simulink model "arm_muscle"  (Simulink 8.1)
settings: Solver=ode3  StartTime=0.0  StopTime=10  FixedStep=1e-2  MaxStep=1e-2  RelTol=1e-3
values from neighbouring files (symbols this model uses):
  c = 0.05    [muscleParams.m]    (also in nms_model_MechInit.m)
  c_jointstop = 0.3 / (pi/180)    (= 17.1887338539)    [muscleParams.m]    (also in nms_model_MechInit.m)
  eref = 0.04    [muscleParams.m]    (also in nms_model_MechInit.m)
  FmaxVAS = 300    [muscleParams.m]    (also in nms_model_MechInit.m = 6000)
  g = 9.81    [init_param.m]    (also in nms_model_MechInit.m)
  K = 5    [muscleParams.m]    (also in nms_model_MechInit.m)
  L1 = 0.28    [init_param.m]
  L2 = 0.32    [init_param.m]
  loptVAS = 0.13    [muscleParams.m]    (also in nms_model_MechInit.m = 0.08)
  lslackVAS = 0.23    [muscleParams.m]    (also in nms_model_MechInit.m)
  m1 = 1.9    [init_param.m]
  N = 1.5    [muscleParams.m]    (also in nms_model_MechInit.m)
  phi23_UpLimit = 155*pi/180    (= 2.70526034059)    [muscleParams.m]    (also in nms_model_MechInit.m = 3.05432619099)
  phimaxVAS = 90*pi/180    (= 1.57079632679)    [muscleParams.m]    (also in nms_model_MechInit.m = 2.87979326579)
  phirefVAS = 60*pi/180    (= 1.0471975512)    [muscleParams.m]    (also in nms_model_MechInit.m = 2.18166156499)
  rhoVAS = 3    [muscleParams.m]    (also in nms_model_MechInit.m = 0.7)
  rVAS = 0.03    [muscleParams.m]    (also in nms_model_MechInit.m = 0.06)
  s = orProblemSendCommand(['LoadIKFastSolver robot Translation3D'],probid)    [init.m]
  tau = 0.01    [muscleParams.m]    (also in nms_model_MechInit.m)
  vmaxVAS = 12    [muscleParams.m]    (also in nms_model_MechInit.m)
  w = 0.56    [muscleParams.m]    (also in nms_model_MechInit.m)
  w_max_jointstop = 1 * pi/180    (= 0.0174532925199)    [muscleParams.m]    (also in nms_model_MechInit.m)
libraries: mblibv1 x27, simulink x1, simulink_extras x1
settings Model: Creator=hgeyer  LastModifiedBy=icoderaven
settings DataIOCC: SignalLoggingSaveFormat=Dataset
settings DebuggingCC: MultiTaskDSMMsg=warning  MultiTaskCondExecSysMsg=none  FcnCallInpInsideContextMsg=EnableAllAsWarning  StrictBusMsg=None
settings RTWCC: IncludeERTFirstTime=on
settings GRTTargetCC: CombineOutputUpdateFcns=on  GRTInterface=off
settings SimMechanicsCC: VisOnUpdateDiagram=on  VisDuringSimulation=on
settings ConfigurationSet: Description=SimMechanics 2G

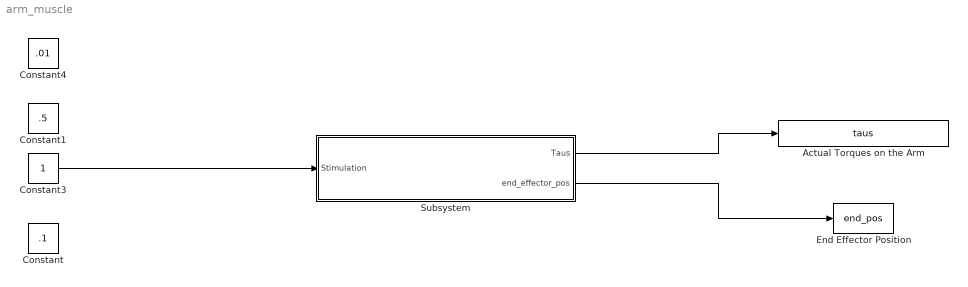
== system arm_muscle ==
  Actual Torques on the Arm : ToWorkspace  VariableName=taus  SampleTime=-1  SaveFormat=Timeseries
  Constant : Constant  Value=.1
  Constant1 : Constant  Value=.5
  Constant3 : Constant
  Constant4 : Constant  Value=.01
  End Effector Position : ToWorkspace  VariableName=end_pos  SampleTime=-1  SaveFormat=Timeseries
  Subsystem : Subsystem
  wires:
  Subsystem/1(Taus) -> Actual Torques on the Arm/1
  Subsystem/2(end_effector_pos) -> End Effector Position/1
  Constant3/1 -> Subsystem/1(Stimulation)

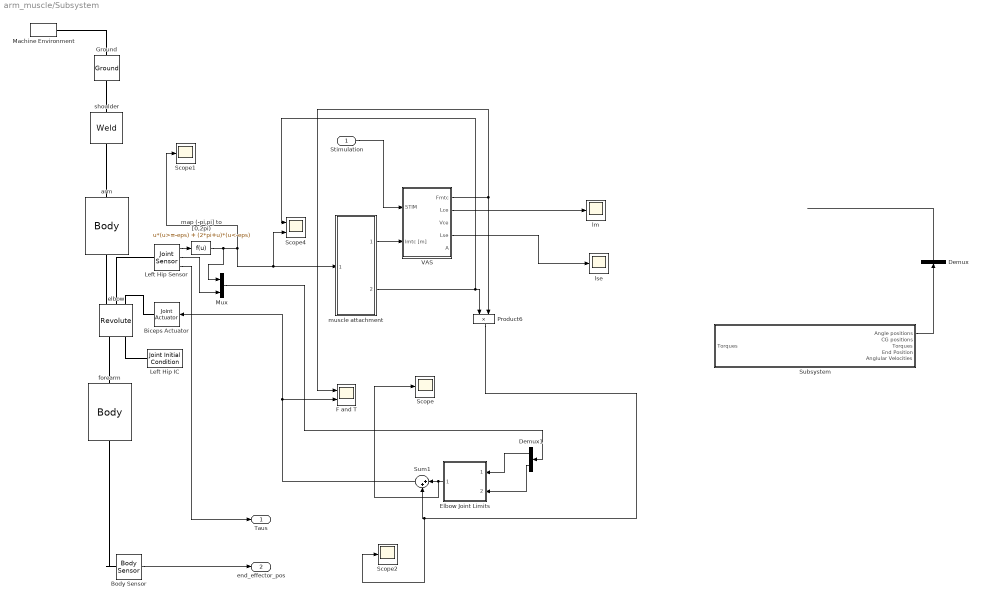
== system arm_muscle/Subsystem ==
  Stimulation : Inport
  Biceps Actuator : mblibv1/Sensors &  Actuators/Joint Actuator  UpdateFromCAD=off  PhysicalDomain=Mechanical  PortType=blob  ActuationStyle=Force  AngleUnits=deg  ArcVelocityUnits=deg/s  ArcAccelerationUnits=deg/s^2  CoordPositionUnits=m  VelocityUnits=m/s  AccelerationUnits=m/s^2  ForceUnits=N  TorqueUnits=N-m  ActiveIO=on  Width=1  DialogClass=MechanicalActuatorBlock  Primitive=R1  ReferenceFrame=Absolute (INERTIAL)
  Body Sensor : mblibv1/Sensors &  Actuators/Body Sensor  UpdateFromCAD=off  PhysicalDomain=Mechanical  PortType=blob  Muxed=on  Pose=off  Angle=on  AngleUnits=deg  ArcVelocity=off  ArcVelocityUnits=deg/s  ArcAcceleration=off  ArcAccelerationUnits=deg/s^2  CoordPosition=on  CoordPositionUnits=m  Velocity=off  VelocityUnits=m/s  Acceleration=off  AccelerationUnits=m/s^2  Quaternion=on  QuaternionDT=off  QuaternionDDT=off  QuaternionUnits=off  OutputVector=[1]  ActiveIO=on  Width=3  DialogClass=MechanicalSensorBlock  ReferenceFrame=Absolute (World)
  Demux : Demux  Outputs=3
  Demux1 : Demux  Outputs=2
  Elbow Joint Limits : Subsystem
  F and T : Scope  NumInputPorts=2
      settings: YMin=-5~-5  YMax=5~5  SaveName=ScopeData3
  Ground : mblibv1/Bodies/Ground  UpdateFromCAD=off  LeftPortType=env  RightPortType=workingframe  PhysicalDomain=Mechanical  DialogClass=GroundBlock  CoordPosition=[0 0 0]  CoordPositionUnits=m  StateVectorMgrId=3  MachineId=[4 0]  ShowEnvPort=on
  Left Hip Sensor : mblibv1/Sensors &  Actuators/Joint Sensor  UpdateFromCAD=off  PhysicalDomain=Mechanical  PortType=blob  Muxed=off  Pose=off  Angle=on  AngleUnits=rad  ArcVelocity=on  ArcVelocityUnits=rad/s  ArcAcceleration=off  ArcAccelerationUnits=deg/s^2  CoordPosition=on  CoordPositionUnits=m  Velocity=on  VelocityUnits=m/s  Acceleration=off  AccelerationUnits=m/s^2  Quaternion=on  QuaternionDT=off  QuaternionDDT=off  QuaternionUnits=off  OutputVector=[ 1 1 ]  ActiveIO=on  Width=3  DialogClass=MechanicalSensorBlock  Primitive=R1  Force=off  ForceUnits=N  Torque=on  TorqueUnits=N*m  ReferenceFrame=Absolute (INERTIAL)  ReactionSensedSide=Base  ReactionReferenceFrame=Absolute (World)  ReactionForce=off  ReactionForceUnits=N  ReactionMoment=off  ReactionMomentUnits=N*m
  Left Hip IC : mblibv1/Sensors &  Actuators/Joint Initial Condition  UpdateFromCAD=off  LeftPortType=blob  RightPortType=blob  PhysicalDomain=mechanical  DialogClass=InitialConditionBlock  InitialConditions=P1$false$0$m$rad$0$m/s$rad/s#P2$false$0$m$rad$0$m/s$rad/s#P3$false$0$m$rad$0$m/s$rad/s#R1$false$90*pi/180$m$rad$0$m/s$rad/s#R2$false$0$m$rad$0$m/s$rad/s#R3$false$0$m$rad$0$m/s$rad/s#S$false$0$m$rad$0$m/s$rad/s  P1PIC=0  P1VIC=0  P2PIC=0  P2VIC=0  P3PIC=0  P3VIC=0  R1PIC=0  R1VIC=0  R2PIC=0  R2VIC=0  R3PIC=0  R3VIC=0  SPIC=0  SVIC=0
  Machine Environment : mblibv1/Bodies/Machine Environment  PortType=env  PhysicalDomain=Mechanical  DialogTemplateClass=MECH.MachineEnvironment  SyncWhenCopied=off  Gravity=[0 -g 0]  GravityUnits=m/s^2  GravityAsSignal=off  Dimensionality=Auto-detect  AnalysisType=Forward dynamics  LinearAssemblyTolerance=1e-3  LinearAssemblyToleranceUnits=m  AngularAssemblyTolerance=1e-3  AngularAssemblyToleranceUnits=rad  ConstraintSolverType=Stabilizing  ConstraintRelTolerance=1e-4  ConstraintAbsTolerance=1e-4  UseRobustSingularityHandling=off  RedundancyAnalysisToleranceType=Automatically select tolerance  RedundancyAnalysisTolerance=1e-14  StatePerturbationType=Fixed  PerturbationSize=1e-5  VisualizeMachine=on  BodyVisualizationType=Use model default body geometries  BodyColorSelMode=Use model default  DefaultBodyColor=[1 0 0]
  Mux : Mux  Inputs=2
  Product6 : Product  RndMeth=Zero
  Scope : Scope
  Scope1 : Scope
      settings: YMin=0.588  YMax=0.5895
  Scope2 : Scope
      settings: YMin=0.588  YMax=0.5895  SaveName=ScopeData2
  Scope4 : Scope  NumInputPorts=2
      settings: YMin=-5~-5  YMax=5~5  SaveName=ScopeData4
  Subsystem : Subsystem
  Sum1 : Sum  Inputs=|++
  VAS : Subsystem
  arm : mblibv1/Bodies/Body  LConnTagsString=CS1  RConnTagsString=CS2  UpdateFromCAD=off  DialogClass=MechanicalBodyBlock  Mass=m1  MassUnits=kg  InertiaUnits=kg*m^2  Inertia=eye(3)  Shape=Cylinder  ShapeDims=[1 1]  ShapeUnits=m  ShapeUse=false  Density=1  DensityUnits=kg/m^3  DensityUse=false  GraphicsMode=MACHINE_DEFAULT  BodyColorSelMode=MACHINE_DEFAULT  BodyColor=[1 0 0]  AttachedToCS=CG  CG=Left$CG$[0 -L1 0]$CS1$CS1$m$[0 0 0]$Euler X-Y-Z$deg$WORLD$false$none  WorkingFrames=Left$CS1$[0 0 0]$Adjoining$Adjoining$m$[0 0 0]$Euler X-Y-Z$deg$WORLD$true$none#Right$CS2$[0 -L1 0]$CS1$CS1$m$[0 0 0]$Euler X-Y-Z$deg$WORLD$true$none  CGPos=[0 -L1 0]  CGRot=[0 0 0]  CS0Pos=[]  CS0Rot=[]  CS1Pos=[0 0 0]  CS1Rot=[0 0 0]  CS2Pos=[0 -L1 0]  CS2Rot=[0 0 0]  CS3Pos=[]  CS3Rot=[]  CS4Pos=[]  CS4Rot=[]  CS5Pos=[]  CS5Rot=[]  CS6Pos=[]  CS6Rot=[]  CS7Pos=[]  CS7Rot=[]  CS8Pos=[]  CS8Rot=[]  CS9Pos=[]  CS9Rot=[]  CS10Pos=[]  CS10Rot=[]  CS11Pos=[]  CS11Rot=[]  CS12Pos=[]  CS12Rot=[]  CS13Pos=[]  CS13Rot=[]  CS14Pos=[]  CS14Rot=[]  CS15Pos=[]  CS15Rot=[]  CS16Pos=[]  CS16Rot=[]  CS17Pos=[]  CS17Rot=[]  CS18Pos=[]  CS18Rot=[]  CS19Pos=[]  CS19Rot=[]  CS20Pos=[]  CS20Rot=[]
  elbow : mblibv1/Joints/Revolute  LConnTagsString=__newl0|SA1|SA2  RConnTagsString=__newr0|SA1  UpdateFromCAD=off  NumSAPorts=3  CutJoint=off  MarkAsCut=off  Primitives=prismatic  PrimitiveProps=R1$World$[0 0 1]$revolute  DialogClass=JointBlock  R1Axis=[0 0 1]
  forearm : mblibv1/Bodies/Body  LConnTagsString=CS1  RConnTagsString=CS2  UpdateFromCAD=off  DialogClass=MechanicalBodyBlock  Mass=3  MassUnits=kg  InertiaUnits=kg*m^2  Inertia=eye(3)  Shape=Cylinder  ShapeDims=[1 1]  ShapeUnits=m  ShapeUse=false  Density=1  DensityUnits=kg/m^3  DensityUse=false  GraphicsMode=MACHINE_DEFAULT  BodyColorSelMode=MACHINE_DEFAULT  BodyColor=[1 0 0]  AttachedToCS=CG  CG=Left$CG$[0 -L2 0]$CS1$CS1$m$[0 0 0]$Euler X-Y-Z$deg$WORLD$false$none  WorkingFrames=Left$CS1$[0 0 0]$Adjoining$Adjoining$m$[0 0 0]$Euler X-Y-Z$deg$WORLD$true$none#Right$CS2$[0 -L2 0]$CS1$CS1$m$[0 0 0]$Euler X-Y-Z$deg$WORLD$true$none  CGPos=[0 -L2 0]  CGRot=[0 0 0]  CS0Pos=[]  CS0Rot=[]  CS1Pos=[0 0 0]  CS1Rot=[0 0 0]  CS2Pos=[0 -L2 0]  CS2Rot=[0 0 0]  CS3Pos=[]  CS3Rot=[]  CS4Pos=[]  CS4Rot=[]  CS5Pos=[]  CS5Rot=[]  CS6Pos=[]  CS6Rot=[]  CS7Pos=[]  CS7Rot=[]  CS8Pos=[]  CS8Rot=[]  CS9Pos=[]  CS9Rot=[]  CS10Pos=[]  CS10Rot=[]  CS11Pos=[]  CS11Rot=[]  CS12Pos=[]  CS12Rot=[]  CS13Pos=[]  CS13Rot=[]  CS14Pos=[]  CS14Rot=[]  CS15Pos=[]  CS15Rot=[]  CS16Pos=[]  CS16Rot=[]  CS17Pos=[]  CS17Rot=[]  CS18Pos=[]  CS18Rot=[]  CS19Pos=[]  CS19Rot=[]  CS20Pos=[]  CS20Rot=[]
  lm : Scope
      settings: SaveName=ScopeData5
  "lse  " : Scope
      settings: TimeRange=10  SaveName=ScopeData8
  map (-pi,pi] to [0,2pi) : Fcn  Expr=u*(u>=-eps) + (2*pi+u)*(u<-eps)
  muscle attachment : Subsystem
  shoulder : mblibv1/Joints/Weld  LConnTagsString=__newl0  RConnTagsString=__newr0  UpdateFromCAD=off  NumSAPorts=0  CutJoint=off  MarkAsCut=off  Primitives=weld  PrimitiveProps=W$WORLD$[0 0 0]$weld  DialogClass=JointBlock  WAxis=[0 0 0]
  Taus : Outport
  end_effector_pos : Outport  Port=2
  wires:
  Left Hip Sensor/1 -> map (-pi,pi] to [0,2pi)/1
  muscle attachment/1(lmtu [m]) -> VAS/2(lmtc [m])
  VAS/1(Fmtc) -> F and T/1, Product6/2
  muscle attachment/2(lever [m]) -> Scope4/1, Product6/1
  Stimulation/1 -> VAS/1(STIM)
  Elbow Joint Limits/1(M_stop [Nm]) -> Scope/1, Sum1/1
  Demux1/1 -> Elbow Joint Limits/1(phi [rad])
  Demux1/2 -> Elbow Joint Limits/2(dphi [rad/s])
  Mux/1 -> Demux1/1
  Sum1/1 -> Biceps Actuator/1, F and T/2
  Product6/1 -> Scope2/1, Sum1/2
  Left Hip Sensor/2 -> Mux/2
  map (-pi,pi] to [0,2pi)/1 -> Mux/1, Scope4/2, muscle attachment/1(phi23 [rad]), Scope1/1
  Left Hip Sensor/3 -> Taus/1
  Body Sensor/1 -> end_effector_pos/1
  VAS/2(Lce) -> lm/1
  VAS/4(Lse) -> "lse  "/1
  Subsystem/1(Angle positions) -> Demux/1
  Demux/2 -> ?
  connections:
  Left Hip Sensor/LConn1 -- elbow/LConn2
  Biceps Actuator/RConn1 -- elbow/LConn3
  Machine Environment/RConn1 -- Ground/LConn1
  Ground/RConn1 -- shoulder/LConn1
  shoulder/RConn1 -- arm/LConn1
  arm/RConn1 -- elbow/LConn1
  elbow/RConn1 -- forearm/LConn1
  Left Hip IC/RConn1 -- elbow/RConn2
  Body Sensor/LConn1 -- forearm/RConn1

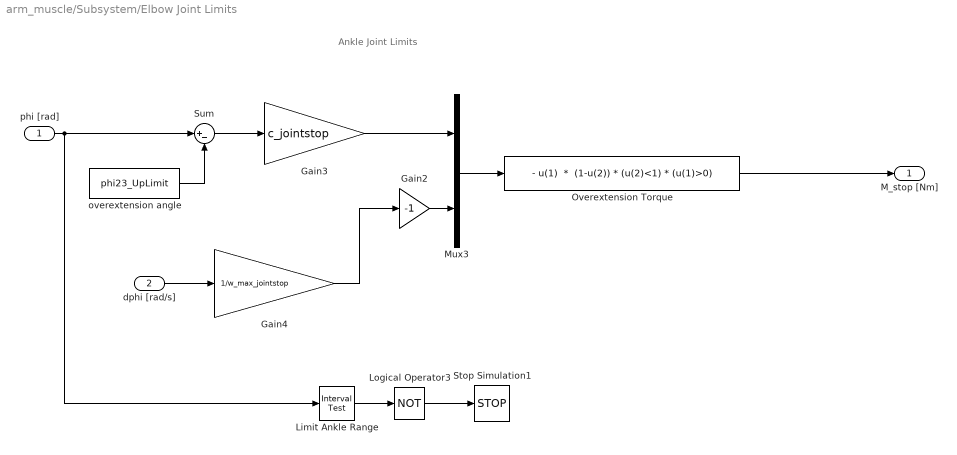
== system arm_muscle/Subsystem/Elbow Joint Limits ==
  note: Ankle Joint Limits
  phi [rad] : Inport
  dphi [rad/s] : Inport  Port=2
  Gain2 : Gain  Gain=-1
  Gain3 : Gain  Gain=c_jointstop
  Gain4 : Gain  Gain=1/w_max_jointstop
  Limit Ankle Range : simulink/Logic and Bit Operations/Interval Test  IntervalClosedRight=on  uplimit=160*pi/180  IntervalClosedLeft=on  lowlimit=0*pi/180  OutDataTypeStr=boolean
  Logical Operator3 : Logic  Operator=NOT  AllPortsSameDT=off  OutDataTypeStr=boolean
  Mux3 : Mux  Inputs=2
  Overextension Torque : Fcn  Expr="- u(1)  *  (1-u(2)) * (u(2)<1) * (u(1)>0)"
  Stop Simulation1 : Stop
  Sum : Sum  Inputs=|+-
  overextension angle : Constant  Value=phi23_UpLimit
  M_stop [Nm] : Outport
  wires:
  Mux3/1 -> Overextension Torque/1
  Gain3/1 -> Mux3/1
  dphi [rad/s]/1 -> Gain4/1
  overextension angle/1 -> Sum/2
  phi [rad]/1 -> Sum/1, Limit Ankle Range/1
  Sum/1 -> Gain3/1
  Gain4/1 -> Gain2/1
  Gain2/1 -> Mux3/2
  Overextension Torque/1 -> M_stop [Nm]/1
  Limit Ankle Range/1 -> Logical Operator3/1
  Logical Operator3/1 -> Stop Simulation1/1

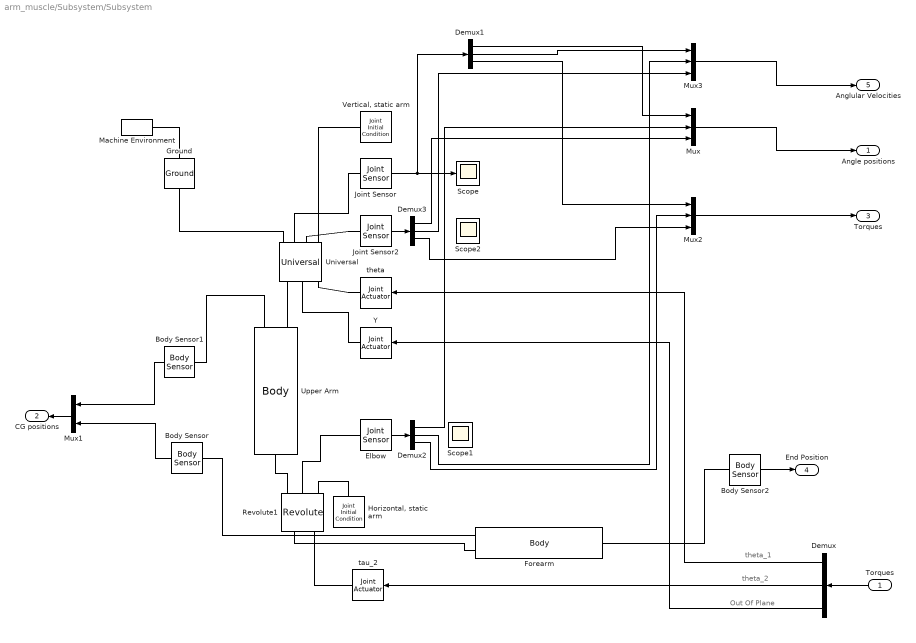
== system arm_muscle/Subsystem/Subsystem ==
  note: theta_2
  note: theta_1
  note: Out Of Plane
  "Torques " : Inport
  Body Sensor : mblibv1/Sensors &  Actuators/Body Sensor  UpdateFromCAD=off  PhysicalDomain=Mechanical  PortType=blob  Muxed=on  Pose=off  Angle=on  AngleUnits=deg  ArcVelocity=off  ArcVelocityUnits=deg/s  ArcAcceleration=off  ArcAccelerationUnits=deg/s^2  CoordPosition=on  CoordPositionUnits=m  Velocity=off  VelocityUnits=m/s  Acceleration=off  AccelerationUnits=m/s^2  Quaternion=on  QuaternionDT=off  QuaternionDDT=off  QuaternionUnits=off  OutputVector=[1]  ActiveIO=off  Width=3  DialogClass=MechanicalSensorBlock  ReferenceFrame=Absolute (World)
  Body Sensor1 : mblibv1/Sensors &  Actuators/Body Sensor  UpdateFromCAD=off  PhysicalDomain=Mechanical  PortType=blob  Muxed=on  Pose=off  Angle=on  AngleUnits=deg  ArcVelocity=off  ArcVelocityUnits=deg/s  ArcAcceleration=off  ArcAccelerationUnits=deg/s^2  CoordPosition=on  CoordPositionUnits=m  Velocity=off  VelocityUnits=m/s  Acceleration=off  AccelerationUnits=m/s^2  Quaternion=on  QuaternionDT=off  QuaternionDDT=off  QuaternionUnits=off  OutputVector=[1]  ActiveIO=off  Width=3  DialogClass=MechanicalSensorBlock  ReferenceFrame=Absolute (World)
  Body Sensor2 : mblibv1/Sensors &  Actuators/Body Sensor  UpdateFromCAD=off  PhysicalDomain=Mechanical  PortType=blob  Muxed=on  Pose=off  Angle=on  AngleUnits=deg  ArcVelocity=off  ArcVelocityUnits=deg/s  ArcAcceleration=off  ArcAccelerationUnits=deg/s^2  CoordPosition=on  CoordPositionUnits=m  Velocity=off  VelocityUnits=m/s  Acceleration=off  AccelerationUnits=m/s^2  Quaternion=on  QuaternionDT=off  QuaternionDDT=off  QuaternionUnits=off  OutputVector=[1]  ActiveIO=off  Width=3  DialogClass=MechanicalSensorBlock  ReferenceFrame=Absolute (World)
  Demux{,1..3} (4 alike) : Demux  Outputs=3
  Elbow : mblibv1/Sensors &  Actuators/Joint Sensor  UpdateFromCAD=off  PhysicalDomain=Mechanical  PortType=blob  Muxed=on  Pose=off  Angle=on  AngleUnits=rad  ArcVelocity=on  ArcVelocityUnits=rad/s  ArcAcceleration=off  ArcAccelerationUnits=deg/s^2  CoordPosition=on  CoordPositionUnits=m  Velocity=off  VelocityUnits=m/s  Acceleration=off  AccelerationUnits=m/s^2  Quaternion=on  QuaternionDT=off  QuaternionDDT=off  QuaternionUnits=off  OutputVector=[1]  ActiveIO=off  Width=3  DialogClass=MechanicalSensorBlock  Primitive=R1  Force=off  ForceUnits=N  Torque=on  TorqueUnits=N*m  ReferenceFrame=Absolute (World)  ReactionSensedSide=Base  ReactionReferenceFrame=Absolute (World)  ReactionForce=off  ReactionForceUnits=N  ReactionMoment=off  ReactionMomentUnits=N*m
  Forearm : mblibv1/Bodies/Body  LConnTagsString=CG|CS1  RConnTagsString=CS2  UpdateFromCAD=off  DialogClass=MechanicalBodyBlock  Mass=1  MassUnits=kg  InertiaUnits=kg*m^2  Inertia=eye(3)  Shape=Cylinder  ShapeDims=[1 1]  ShapeUnits=m  ShapeUse=false  Density=1  DensityUnits=kg/m^3  DensityUse=false  GraphicsMode=MACHINE_DEFAULT  BodyColorSelMode=MACHINE_DEFAULT  BodyColor=[1 0 0]  AttachedToCS=CG  CG=Left$CG$[0 -L2/2 0]$CS1$CS1$m$[0 0 0]$Euler X-Y-Z$deg$WORLD$true$none  WorkingFrames=Left$CS1$[0 0 0]$Adjoining$Adjoining$m$[0 0 0]$Euler X-Y-Z$deg$WORLD$true$none#Right$CS2$[0 -L2 0]$CS1$CS1$m$[0 0 0]$Euler X-Y-Z$deg$WORLD$true$none  CGPos=[0 -L2/2 0]  CGRot=[0 0 0]  CS0Pos=[]  CS0Rot=[]  CS1Pos=[0 0 0]  CS1Rot=[0 0 0]  CS2Pos=[0 -L2 0]  CS2Rot=[0 0 0]  CS3Pos=[]  CS3Rot=[]  CS4Pos=[]  CS4Rot=[]  CS5Pos=[]  CS5Rot=[]  CS6Pos=[]  CS6Rot=[]  CS7Pos=[]  CS7Rot=[]  CS8Pos=[]  CS8Rot=[]  CS9Pos=[]  CS9Rot=[]  CS10Pos=[]  CS10Rot=[]  CS11Pos=[]  CS11Rot=[]  CS12Pos=[]  CS12Rot=[]  CS13Pos=[]  CS13Rot=[]  CS14Pos=[]  CS14Rot=[]  CS15Pos=[]  CS15Rot=[]  CS16Pos=[]  CS16Rot=[]  CS17Pos=[]  CS17Rot=[]  CS18Pos=[]  CS18Rot=[]  CS19Pos=[]  CS19Rot=[]  CS20Pos=[]  CS20Rot=[]
  Ground : mblibv1/Bodies/Ground  UpdateFromCAD=off  LeftPortType=env  RightPortType=workingframe  PhysicalDomain=Mechanical  DialogClass=GroundBlock  CoordPosition=[0 0 0]  CoordPositionUnits=m  StateVectorMgrId=-1  MachineId=[0 0]  ShowEnvPort=on
  "Horizontal, static arm" : mblibv1/Sensors &  Actuators/Joint Initial Condition  UpdateFromCAD=off  LeftPortType=blob  RightPortType=blob  PhysicalDomain=mechanical  DialogClass=InitialConditionBlock  InitialConditions=P1$false$0$m$deg$0$m/s$deg/s#P2$false$0$m$deg$0$m/s$deg/s#P3$false$0$m$deg$0$m/s$deg/s#R1$false$0$m$deg$0$m/s$deg/s#R2$false$0$m$deg$0$m/s$deg/s#R3$false$0$m$deg$0$m/s$deg/s#S$false$0$m$deg$0$m/s$deg/s  P1PIC=0  P1VIC=0  P2PIC=0  P2VIC=0  P3PIC=0  P3VIC=0  R1PIC=0  R1VIC=0  R2PIC=0  R2VIC=0  R3PIC=0  R3VIC=0  SPIC=0  SVIC=0
  Joint Sensor : mblibv1/Sensors &  Actuators/Joint Sensor  UpdateFromCAD=off  PhysicalDomain=Mechanical  PortType=blob  Muxed=on  Pose=off  Angle=on  AngleUnits=rad  ArcVelocity=on  ArcVelocityUnits=rad/s  ArcAcceleration=off  ArcAccelerationUnits=deg/s^2  CoordPosition=on  CoordPositionUnits=m  Velocity=off  VelocityUnits=m/s  Acceleration=off  AccelerationUnits=m/s^2  Quaternion=on  QuaternionDT=off  QuaternionDDT=off  QuaternionUnits=off  OutputVector=[1]  ActiveIO=off  Width=3  DialogClass=MechanicalSensorBlock  Primitive=R1  Force=off  ForceUnits=N  Torque=on  TorqueUnits=N*m  ReferenceFrame=Absolute (World)  ReactionSensedSide=Base  ReactionReferenceFrame=Absolute (World)  ReactionForce=off  ReactionForceUnits=N  ReactionMoment=off  ReactionMomentUnits=N*m
  Joint Sensor2 : mblibv1/Sensors &  Actuators/Joint Sensor  UpdateFromCAD=off  PhysicalDomain=Mechanical  PortType=blob  Muxed=on  Pose=off  Angle=on  AngleUnits=rad  ArcVelocity=on  ArcVelocityUnits=rad/s  ArcAcceleration=off  ArcAccelerationUnits=deg/s^2  CoordPosition=on  CoordPositionUnits=m  Velocity=off  VelocityUnits=m/s  Acceleration=off  AccelerationUnits=m/s^2  Quaternion=on  QuaternionDT=off  QuaternionDDT=off  QuaternionUnits=off  OutputVector=[1]  ActiveIO=off  Width=3  DialogClass=MechanicalSensorBlock  Primitive=R2  Force=off  ForceUnits=N  Torque=on  TorqueUnits=N*m  ReferenceFrame=Absolute (World)  ReactionSensedSide=Base  ReactionReferenceFrame=Absolute (World)  ReactionForce=off  ReactionForceUnits=N  ReactionMoment=off  ReactionMomentUnits=N*m
  Machine Environment : mblibv1/Bodies/Machine Environment  PortType=env  PhysicalDomain=Mechanical  DialogTemplateClass=MECH.MachineEnvironment  SyncWhenCopied=off  Gravity=[0 -g 0]  GravityUnits=m/s^2  GravityAsSignal=off  Dimensionality=Auto-detect  AnalysisType=Forward dynamics  LinearAssemblyTolerance=1e-3  LinearAssemblyToleranceUnits=m  AngularAssemblyTolerance=1e-3  AngularAssemblyToleranceUnits=rad  ConstraintSolverType=Stabilizing  ConstraintRelTolerance=1e-4  ConstraintAbsTolerance=1e-4  UseRobustSingularityHandling=off  RedundancyAnalysisToleranceType=Automatically select tolerance  RedundancyAnalysisTolerance=1e-14  StatePerturbationType=Fixed  PerturbationSize=1e-5  VisualizeMachine=on  BodyVisualizationType=Use model default body geometries  BodyColorSelMode=Use model default  DefaultBodyColor=[1 0 0]
  Mux : Mux  Inputs=3
  Mux1 : Mux  Inputs=2
  Mux2 : Mux  Inputs=3
  Mux3 : Mux  Inputs=3
  Revolute1 : mblibv1/Joints/Revolute  LConnTagsString=__newl0|SA1|SA2  RConnTagsString=__newr0|SA1  UpdateFromCAD=off  NumSAPorts=3  CutJoint=off  MarkAsCut=off  Primitives=prismatic  PrimitiveProps=R1$World$[0 0 1]$revolute  DialogClass=JointBlock  R1Axis=[0 0 1]
  Scope : Scope
  Scope1 : Scope
  Scope2 : Scope
      settings: SaveName=ScopeData2
  Universal : mblibv1/Joints/Universal  LConnTagsString=__newl0|SA1|SA2|SA3  RConnTagsString=__newr0|SA1|SA2  UpdateFromCAD=off  NumSAPorts=5  CutJoint=off  MarkAsCut=off  Primitives=prismatic  PrimitiveProps=R1$World$[0 0 1]$revolute#R2$World$[1 0 0]$revolute  DialogClass=JointBlock  R1Axis=[0 0 1]  R2Axis=[1 0 0]
  Upper Arm : mblibv1/Bodies/Body  LConnTagsString=CG|CS1  RConnTagsString=CS2  UpdateFromCAD=off  DialogClass=MechanicalBodyBlock  Mass=1  MassUnits=kg  InertiaUnits=kg*m^2  Inertia=eye(3)  Shape=Cylinder  ShapeDims=[1 1]  ShapeUnits=m  ShapeUse=false  Density=1  DensityUnits=kg/m^3  DensityUse=false  GraphicsMode=MACHINE_DEFAULT  BodyColorSelMode=MACHINE_DEFAULT  BodyColor=[1 0 0]  AttachedToCS=CG  CG=Left$CG$[0 -L1/2 0]$CS1$CS1$m$[0 0 0]$Euler X-Y-Z$deg$WORLD$true$none  WorkingFrames=Left$CS1$[0 0 0]$World$World$m$[0 0 0]$Euler X-Y-Z$deg$WORLD$true$none#Right$CS2$[0 -L1 0]$CS1$CS1$m$[0 0 0]$Euler X-Y-Z$deg$WORLD$true$none  CGPos=[0 -L1/2 0]  CGRot=[0 0 0]  CS0Pos=[]  CS0Rot=[]  CS1Pos=[0 0 0]  CS1Rot=[0 0 0]  CS2Pos=[0 -L1 0]  CS2Rot=[0 0 0]  CS3Pos=[]  CS3Rot=[]  CS4Pos=[]  CS4Rot=[]  CS5Pos=[]  CS5Rot=[]  CS6Pos=[]  CS6Rot=[]  CS7Pos=[]  CS7Rot=[]  CS8Pos=[]  CS8Rot=[]  CS9Pos=[]  CS9Rot=[]  CS10Pos=[]  CS10Rot=[]  CS11Pos=[]  CS11Rot=[]  CS12Pos=[]  CS12Rot=[]  CS13Pos=[]  CS13Rot=[]  CS14Pos=[]  CS14Rot=[]  CS15Pos=[]  CS15Rot=[]  CS16Pos=[]  CS16Rot=[]  CS17Pos=[]  CS17Rot=[]  CS18Pos=[]  CS18Rot=[]  CS19Pos=[]  CS19Rot=[]  CS20Pos=[]  CS20Rot=[]
  "Vertical, static arm" : mblibv1/Sensors &  Actuators/Joint Initial Condition  UpdateFromCAD=off  LeftPortType=blob  RightPortType=blob  PhysicalDomain=mechanical  DialogClass=InitialConditionBlock  InitialConditions=P1$false$0$m$deg$0$m/s$deg/s#P2$false$0$m$deg$0$m/s$deg/s#P3$false$0$m$deg$0$m/s$deg/s#R1$true$0$m$deg$0$m/s$deg/s#R2$true$0$m$deg$0$m/s$deg/s#R3$false$0$m$deg$0$m/s$deg/s#S$false$0$m$deg$0$m/s$deg/s  P1PIC=0  P1VIC=0  P2PIC=0  P2VIC=0  P3PIC=0  P3VIC=0  R1PIC=0  R1VIC=0  R2PIC=0  R2VIC=0  R3PIC=0  R3VIC=0  SPIC=0  SVIC=0
  Y : mblibv1/Sensors &  Actuators/Joint Actuator  UpdateFromCAD=off  PhysicalDomain=Mechanical  PortType=blob  ActuationStyle=Force  AngleUnits=deg  ArcVelocityUnits=deg/s  ArcAccelerationUnits=deg/s^2  CoordPositionUnits=m  VelocityUnits=m/s  AccelerationUnits=m/s^2  ForceUnits=N  TorqueUnits=N*m  ActiveIO=off  Width=1  DialogClass=MechanicalActuatorBlock  Primitive=R2  ReferenceFrame=Absolute (World)
  tau_2 : mblibv1/Sensors &  Actuators/Joint Actuator  UpdateFromCAD=off  PhysicalDomain=Mechanical  PortType=blob  ActuationStyle=Force  AngleUnits=deg  ArcVelocityUnits=deg/s  ArcAccelerationUnits=deg/s^2  CoordPositionUnits=m  VelocityUnits=m/s  AccelerationUnits=m/s^2  ForceUnits=N  TorqueUnits=N*m  ActiveIO=off  Width=1  DialogClass=MechanicalActuatorBlock  Primitive=R1  ReferenceFrame=Absolute (World)
  theta : mblibv1/Sensors &  Actuators/Joint Actuator  UpdateFromCAD=off  PhysicalDomain=Mechanical  PortType=blob  ActuationStyle=Force  AngleUnits=deg  ArcVelocityUnits=deg/s  ArcAccelerationUnits=deg/s^2  CoordPositionUnits=m  VelocityUnits=m/s  AccelerationUnits=m/s^2  ForceUnits=N  TorqueUnits=N*m  ActiveIO=off  Width=1  DialogClass=MechanicalActuatorBlock  Primitive=R1  ReferenceFrame=Absolute (World)
  Angle positions : Outport
  "CG positions " : Outport  Port=2
  Torques : Outport  Port=3
  End Position : Outport  Port=4
  Anglular Velocities : Outport  Port=5
  wires:
  Demux/3 -> Y/1
  Demux/2 -> tau_2/1
  Joint Sensor/1 -> Demux1/1, Scope/1
  Demux/1 -> theta/1
  "Torques "/1 -> Demux/1
  Mux/1 -> Angle positions/1
  Demux1/1 -> Mux/1
  Demux2/1 -> Mux/2
  Demux3/1 -> Mux/3
  Body Sensor/1 -> Mux1/2
  Mux1/1 -> "CG positions "/1
  Body Sensor1/1 -> Mux1/1
  Mux2/1 -> Torques/1
  Demux2/3 -> Mux2/2
  Demux3/3 -> Mux2/3
  Body Sensor2/1 -> End Position/1
  Demux1/3 -> Mux2/1
  Elbow/1 -> Demux2/1
  Joint Sensor2/1 -> Demux3/1
  Mux3/1 -> Anglular Velocities/1
  Demux1/2 -> Mux3/1
  Demux3/2 -> Mux3/3
  Demux2/2 -> Mux3/2
  connections:
  Universal/LConn1 -- Ground/RConn1
  Universal/RConn1 -- Upper Arm/LConn2
  Revolute1/LConn1 -- Upper Arm/RConn1
  Revolute1/RConn1 -- Forearm/LConn2
  Machine Environment/RConn1 -- Ground/LConn1
  Universal/LConn2 -- Joint Sensor/LConn1
  Universal/RConn2 -- Y/RConn1
  tau_2/RConn1 -- Revolute1/RConn2
  Elbow/LConn1 -- Revolute1/LConn2
  theta/RConn1 -- Universal/RConn3
  Joint Sensor2/LConn1 -- Universal/LConn3
  "Vertical, static arm"/RConn1 -- Universal/LConn4
  Revolute1/LConn3 -- "Horizontal, static arm"/RConn1
  Body Sensor/LConn1 -- Forearm/LConn1
  Upper Arm/LConn1 -- Body Sensor1/LConn1
  Body Sensor2/LConn1 -- Forearm/RConn1

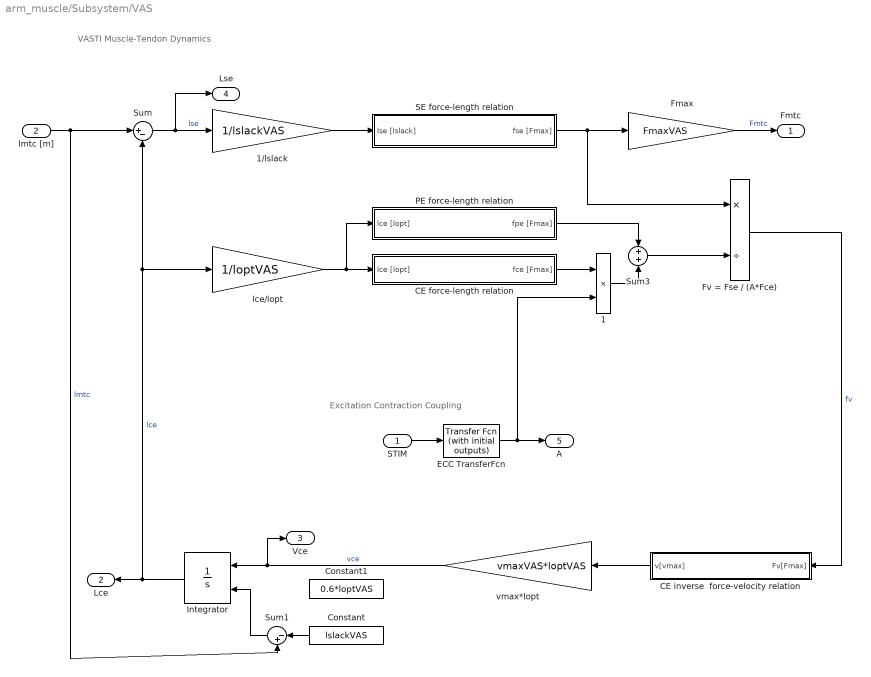
== system arm_muscle/Subsystem/VAS ==
  note: VASTI Muscle-Tendon Dynamics
  note: Excitation Contraction Coupling
  STIM : Inport
  lmtc [m] : Inport  Port=2
  1 : Product  Inputs=**  SaturateOnIntegerOverflow=on  InputSameDT=on  OutDataTypeStr=Inherit: Same as first input
  1/lslack : Gain  Gain=1/lslackVAS  SaturateOnIntegerOverflow=on  OutDataTypeStr=Inherit: Same as input  ParamDataTypeStr=Inherit: Same as input
  CE force-length relation : Subsystem
  CE inverse  force-velocity relation : Subsystem
  Constant : Constant  Value=lslackVAS
  Constant1 : Constant  Value=0.6*loptVAS
  ECC TransferFcn : simulink_extras/Additional Linear/Transfer Fcn (with initial outputs)  N=[1]  D="[tau  1]"  Y0=preA  U0=0
      settings: AttributesFormatString=pre-activation: %<Y0>
  Fmax : Gain  Gain=FmaxVAS  SaturateOnIntegerOverflow=on  OutDataTypeStr=Inherit: Same as input  ParamDataTypeStr=Inherit: Same as input
  Fv = Fse / (A*Fce) : Product  Inputs=*/  SaturateOnIntegerOverflow=on  InputSameDT=on  OutDataTypeStr=Inherit: Same as first input
  Integrator : Integrator  InitialConditionSource=external  LowerSaturationLimit=0.05
  PE force-length relation : Subsystem
  SE force-length relation : Subsystem
  Sum : Sum  Inputs=|+-  SaturateOnIntegerOverflow=on  InputSameDT=on  OutDataTypeStr=Inherit: Same as first input
  Sum1 : Sum  Inputs=|-+  SaturateOnIntegerOverflow=on  InputSameDT=on  OutDataTypeStr=Inherit: Same as first input
  Sum3 : Sum  SaturateOnIntegerOverflow=on  InputSameDT=on  OutDataTypeStr=Inherit: Same as first input
  lce/lopt : Gain  Gain=1/loptVAS  SaturateOnIntegerOverflow=on  OutDataTypeStr=Inherit: Same as input  ParamDataTypeStr=Inherit: Same as input
  vmax*lopt : Gain  Gain=vmaxVAS*loptVAS  SaturateOnIntegerOverflow=on  OutDataTypeStr=Inherit: Same as input  ParamDataTypeStr=Inherit: Same as input
  Fmtc : Outport  InitialOutput=0
  Lce : Outport  Port=2  InitialOutput=0
  Vce : Outport  Port=3  InitialOutput=0
  Lse : Outport  Port=4  InitialOutput=0
  A : Outport  Port=5  InitialOutput=0
  wires:
  Integrator/1 -> Sum/2, lce/lopt/1, Lce/1  "lce"
  Sum/1 -> 1/lslack/1, Lse/1  "lse"
  lce/lopt/1 -> CE force-length relation/1(lce [lopt]), PE force-length relation/1(lce [lopt])
  Fv = Fse / (A*Fce)/1 -> CE inverse  force-velocity relation/1(Fv[Fmax])  "fv"
  vmax*lopt/1 -> Integrator/1, Vce/1  "vce"
  lmtc [m]/1 -> Sum1/2, Sum/1  "lmtc"
  Fmax/1 -> Fmtc/1  "Fmtc"
  1/lslack/1 -> SE force-length relation/1(lse [lslack])
  Constant/1 -> Sum1/1
  CE force-length relation/1(fce [Fmax]) -> 1/1
  SE force-length relation/1(fse [Fmax]) -> Fv = Fse / (A*Fce)/1, Fmax/1
  PE force-length relation/1(fpe [Fmax]) -> Sum3/1
  1/1 -> Sum3/2
  Sum3/1 -> Fv = Fse / (A*Fce)/2
  CE inverse  force-velocity relation/1(v[vmax]) -> vmax*lopt/1
  STIM/1 -> ECC TransferFcn/1
  ECC TransferFcn/1 -> 1/2, A/1
  Sum1/1 -> Integrator/2

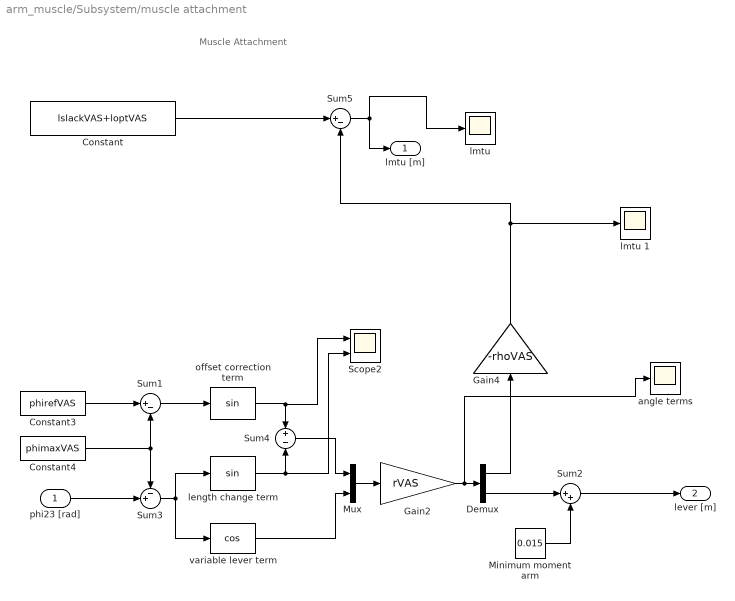
== system arm_muscle/Subsystem/muscle attachment ==
  note: Muscle Attachment
  phi23 [rad] : Inport
  Constant : Constant  Value=lslackVAS+loptVAS
  Constant3 : Constant  Value=phirefVAS
  Constant4 : Constant  Value=phimaxVAS
  Demux : Demux  Outputs=2
  Gain2 : Gain  Gain=rVAS
  Gain4 : Gain  Gain=-rhoVAS
  Minimum moment arm : Constant  Value=0.015
  Mux : Mux  Inputs=2
  Scope2 : Scope  NumInputPorts=2
      settings: YMin=0.906308~-0.9  YMax=0.906308~0.5  SaveName=ScopeData7
  Sum1 : Sum  Inputs=|+-
  Sum2 : Sum  Inputs=|++
  Sum3 : Sum  Inputs=-+|
  Sum4 : Sum  Inputs=+-
  Sum5 : Sum  Inputs=|+-
  "angle terms " : Scope
      settings: TimeRange=8  YMin=-0.03  YMax=0.03  SaveName=ScopeData6
  length change term : Trigonometry
  "lmtu " : Scope
      settings: TimeRange=4  SaveName=ScopeData5
  lmtu 1 : Scope
      settings: SaveName=ScopeData9
  offset correction term : Trigonometry
  variable lever term : Trigonometry  Operator=cos
  lmtu [m] : Outport
  lever [m] : Outport  Port=2
  wires:
  Constant/1 -> Sum5/1
  Sum5/1 -> "lmtu "/1, lmtu [m]/1
  Gain4/1 -> Sum5/2, lmtu 1/1
  phi23 [rad]/1 -> Sum3/2
  Sum3/1 -> variable lever term/1, length change term/1
  Constant4/1 -> Sum3/1, Sum1/2
  Sum1/1 -> offset correction term/1
  Constant3/1 -> Sum1/1
  offset correction term/1 -> Scope2/1, Sum4/1
  length change term/1 -> Sum4/2, Scope2/2
  variable lever term/1 -> Mux/2
  Mux/1 -> Gain2/1
  Gain2/1 -> "angle terms "/1, Demux/1
  Demux/1 -> Gain4/1
  Demux/2 -> Sum2/1
  Minimum moment arm/1 -> Sum2/2
  Sum2/1 -> lever [m]/1
  Sum4/1 -> Mux/1

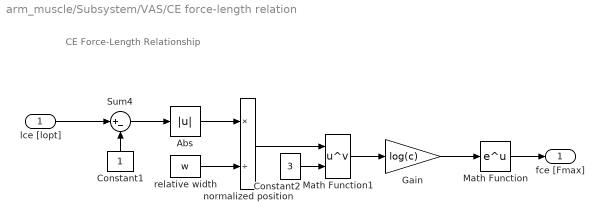
== system arm_muscle/Subsystem/VAS/CE force-length relation ==
  note: CE Force-Length Relationship
  lce [lopt] : Inport
  Abs : Abs
  Constant1 : Constant
  Constant2 : Constant  Value=3
  Gain : Gain  Gain=log(c)
  Math Function : Math  SaturateOnIntegerOverflow=on
  Math Function1 : Math  Operator=pow  SaturateOnIntegerOverflow=on
  Sum4 : Sum  Inputs=|+-  SaturateOnIntegerOverflow=on  InputSameDT=on  OutDataTypeStr=Inherit: Same as first input
  normalized position : Product  Inputs=*/
  relative width : Constant  Value=w
  fce [Fmax] : Outport
  wires:
  lce [lopt]/1 -> Sum4/1
  relative width/1 -> normalized position/2
  Constant1/1 -> Sum4/2
  Sum4/1 -> Abs/1
  Abs/1 -> normalized position/1
  normalized position/1 -> Math Function1/1
  Constant2/1 -> Math Function1/2
  Math Function1/1 -> Gain/1
  Gain/1 -> Math Function/1
  Math Function/1 -> fce [Fmax]/1

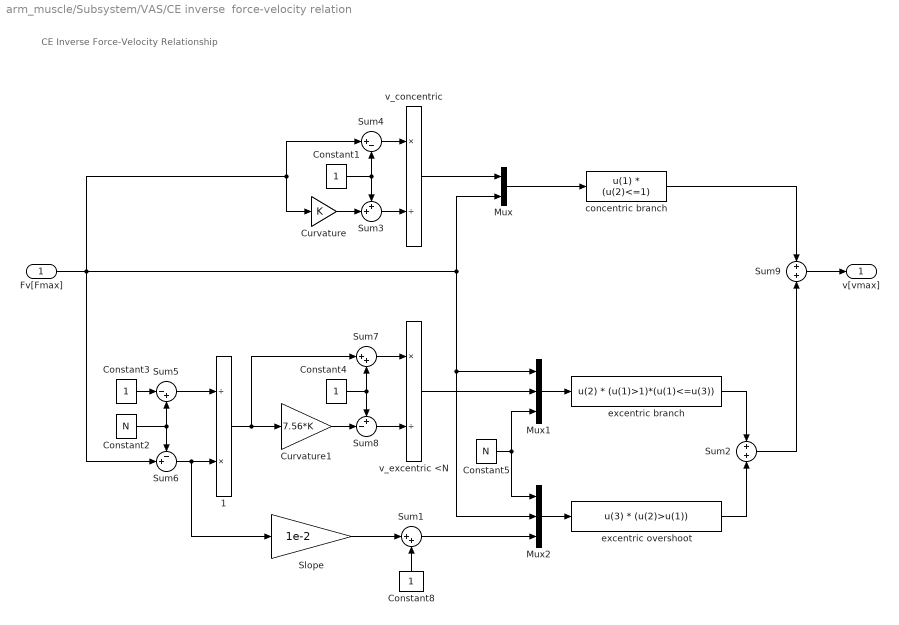
== system arm_muscle/Subsystem/VAS/CE inverse  force-velocity relation ==
  note: CE Inverse Force-Velocity Relationship
  Fv[Fmax] : Inport
  1 : Product  Inputs=/*
  Constant{1,3..4,8} (4 alike) : Constant
  Constant2 : Constant  Value=N
  Constant5 : Constant  Value=N
  Curvature : Gain  Gain=K  SaturateOnIntegerOverflow=on  OutDataTypeStr=Inherit: Same as input  ParamDataTypeStr=Inherit: Same as input
  Curvature1 : Gain  Gain=7.56*K  SaturateOnIntegerOverflow=on  OutDataTypeStr=Inherit: Same as input  ParamDataTypeStr=Inherit: Same as input
  Mux : Mux  Inputs=2
  Mux1 : Mux  Inputs=3
  Mux2 : Mux  Inputs=3
  Slope : Gain  Gain=1e-2  SaturateOnIntegerOverflow=on  OutDataTypeStr=Inherit: Same as input  ParamDataTypeStr=Inherit: Same as input
  Sum1 : Sum  Inputs=|++  SaturateOnIntegerOverflow=on  InputSameDT=on  OutDataTypeStr=Inherit: Same as first input
  Sum2 : Sum  SaturateOnIntegerOverflow=on  InputSameDT=on  OutDataTypeStr=Inherit: Same as first input
  Sum3 : Sum  Inputs=++|  SaturateOnIntegerOverflow=on  InputSameDT=on  OutDataTypeStr=Inherit: Same as first input
  Sum4 : Sum  Inputs=|+-  SaturateOnIntegerOverflow=on  InputSameDT=on  OutDataTypeStr=Inherit: Same as first input
  Sum5 : Sum  Inputs=|-+  SaturateOnIntegerOverflow=on  InputSameDT=on  OutDataTypeStr=Inherit: Same as first input
  Sum6 : Sum  Inputs=-+|  SaturateOnIntegerOverflow=on  InputSameDT=on  OutDataTypeStr=Inherit: Same as first input
  Sum7 : Sum  Inputs=|++  SaturateOnIntegerOverflow=on  InputSameDT=on  OutDataTypeStr=Inherit: Same as first input
  Sum8 : Sum  Inputs=+-|  SaturateOnIntegerOverflow=on  InputSameDT=on  OutDataTypeStr=Inherit: Same as first input
  Sum9 : Sum  SaturateOnIntegerOverflow=on  InputSameDT=on  OutDataTypeStr=Inherit: Same as first input
  concentric branch : Fcn  Expr=u(1) * (u(2)<=1)
  excentric branch : Fcn  Expr=u(2) * (u(1)>1)*(u(1)<=u(3))
  excentric overshoot : Fcn  Expr=u(3) * (u(2)>u(1))
  v_concentric : Product  Inputs=*/
  v_excentric <N : Product  Inputs=*/
  v[vmax] : Outport
  wires:
  Curvature/1 -> Sum3/2
  Constant1/1 -> Sum4/2, Sum3/1
  Sum4/1 -> v_concentric/1
  Sum3/1 -> v_concentric/2
  1/1 -> Sum7/1, Curvature1/1
  Constant4/1 -> Sum7/2, Sum8/1
  Curvature1/1 -> Sum8/2
  Sum8/1 -> v_excentric <N/2
  Sum7/1 -> v_excentric <N/1
  v_concentric/1 -> Mux/1
  Fv[Fmax]/1 -> Sum4/1, Curvature/1, Sum6/2, Mux/2, Mux1/1, Mux2/2
  Sum9/1 -> v[vmax]/1
  Sum2/1 -> Sum9/2
  excentric overshoot/1 -> Sum2/2
  Slope/1 -> Sum1/1
  Constant8/1 -> Sum1/2
  Sum6/1 -> 1/2, Slope/1
  Constant2/1 -> Sum6/1, Sum5/2
  Sum5/1 -> 1/1
  Constant3/1 -> Sum5/1
  Mux/1 -> concentric branch/1
  Mux1/1 -> excentric branch/1
  v_excentric <N/1 -> Mux1/2
  Mux2/1 -> excentric overshoot/1
  concentric branch/1 -> Sum9/1
  excentric branch/1 -> Sum2/1
  Constant5/1 -> Mux1/3, Mux2/1
  Sum1/1 -> Mux2/3

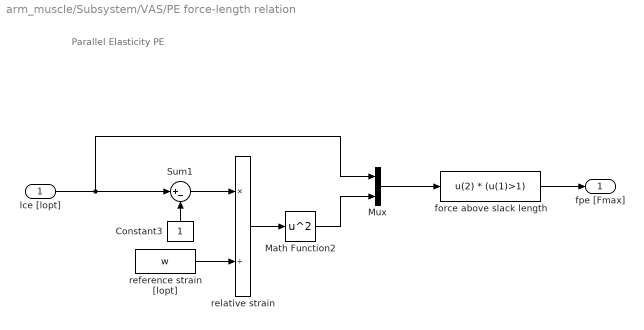
== system arm_muscle/Subsystem/VAS/PE force-length relation ==
  note: Parallel Elasticity PE
  lce [lopt] : Inport
  Constant3 : Constant
  Math Function2 : Math  Operator=square  SaturateOnIntegerOverflow=on
  Mux : Mux  Inputs=2
  Sum1 : Sum  Inputs=|+-  SaturateOnIntegerOverflow=on  InputSameDT=on  OutDataTypeStr=Inherit: Same as first input
  force above slack length : Fcn  Expr=u(2) * (u(1)>1)
  reference strain [lopt] : Constant  Value=w
  relative strain : Product  Inputs=*/
  fpe [Fmax] : Outport
  wires:
  Mux/1 -> force above slack length/1
  lce [lopt]/1 -> Mux/1, Sum1/1
  Constant3/1 -> Sum1/2
  Sum1/1 -> relative strain/1
  reference strain [lopt]/1 -> relative strain/2
  relative strain/1 -> Math Function2/1
  Math Function2/1 -> Mux/2
  force above slack length/1 -> fpe [Fmax]/1

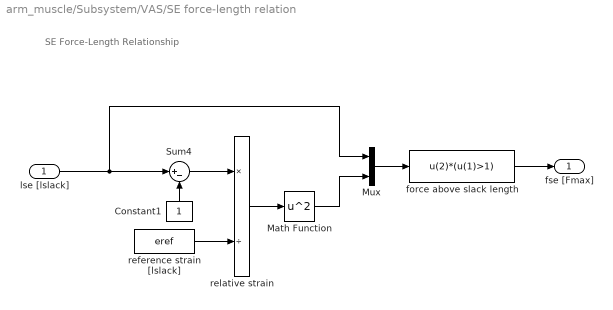
== system arm_muscle/Subsystem/VAS/SE force-length relation ==
  note: SE Force-Length Relationship
  lse [lslack] : Inport
  Constant1 : Constant
  Math Function : Math  Operator=square  SaturateOnIntegerOverflow=on
  Mux : Mux  Inputs=2
  Sum4 : Sum  Inputs=|+-  SaturateOnIntegerOverflow=on  InputSameDT=on  OutDataTypeStr=Inherit: Same as first input
  force above slack length : Fcn  Expr=u(2)*(u(1)>1)
  reference strain [lslack] : Constant  Value=eref
  relative strain : Product  Inputs=*/
  fse [Fmax] : Outport
  wires:
  Mux/1 -> force above slack length/1
  force above slack length/1 -> fse [Fmax]/1
  Math Function/1 -> Mux/2
  lse [lslack]/1 -> Mux/1, Sum4/1
  relative strain/1 -> Math Function/1
  reference strain [lslack]/1 -> relative strain/2
  Sum4/1 -> relative strain/1
  Constant1/1 -> Sum4/2
